simulink model "celcius_to_fahrenheit_testing"  (R2015a)
settings: Solver=ode45  StartTime=0.0  StopTime=10.0  RelTol=1e-3
libraries: simulink x1
settings Model: Creator=USER  LastModifiedBy=USER

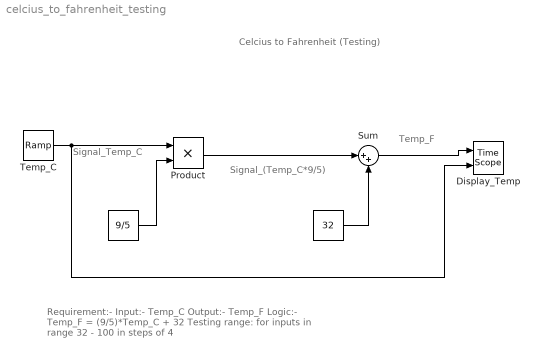
== system celcius_to_fahrenheit_testing ==
  note: Requirement:-
      |
      | Input:- Temp_C
      | Output:- Temp_F
      | Logic:- Temp_F = (9/5)*Temp_C + 32
      | Testing range: for inputs in range 32 - 100 in steps of 4
  note: Temp_F
  note: Signal_(Temp_C*9/5)
  note: Signal_Temp_C
  note: Celcius to Fahrenheit (Testing)
  " " : Constant  Value=9/5
  " " : Constant  Value=32
  Display_Temp : TimeScope  NumInputPorts=2
  Product : Product
  Sum : Sum  Inputs=|++
  Temp_C : simulink/Sources/Ramp  slope=4  start=0  X0=0
  wires:
  Temp_C/1 -> Display_Temp/2, Product/1
  " "/1 -> Product/2
  Product/1 -> Sum/1
  " "/1 -> Sum/2
  Sum/1 -> Display_Temp/1
